simulink model "BasicACCTest"  (R2014a)
settings: Solver=ode45  StartTime=0.0  StopTime=10.0  RelTol=1e-3
values from neighbouring files (symbols this model uses):
  Engine =     [ECR1.mat]    (also in GenPT001.mat)
  Trans =     [ECR1.mat]    (also in GenPT001.mat)
libraries: simulink x2
settings Model: Creator=swami  LastModifiedBy=swami

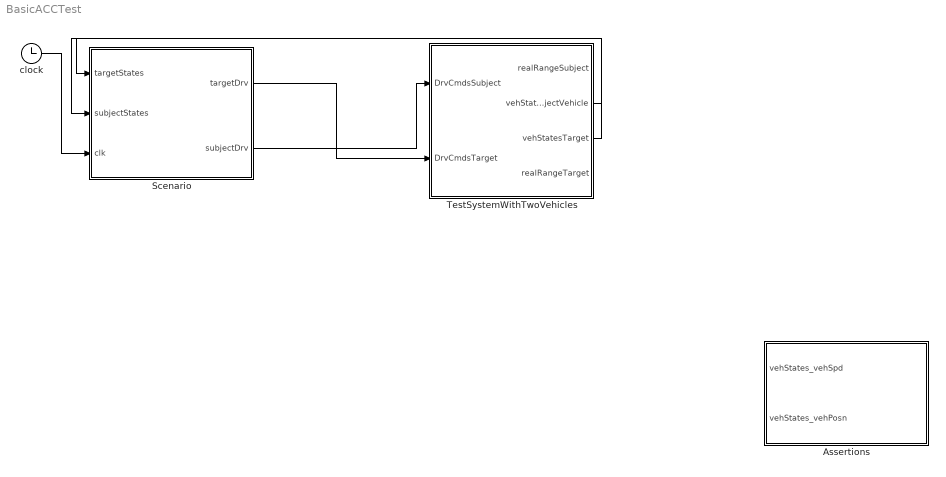
== system BasicACCTest ==
  Assertions : Subsystem
  Scenario : Stateflow chart  TreatAsAtomicUnit=on
  TestSystemWithTwoVehicles : Subsystem
  clock : Clock
  wires:
  Scenario/1(targetDrv) -> TestSystemWithTwoVehicles/2(DrvCmdsTarget)
  Scenario/2(subjectDrv) -> TestSystemWithTwoVehicles/1(DrvCmdsSubject)
  TestSystemWithTwoVehicles/3(vehStatesTarget) -> Scenario/1(targetStates)
  TestSystemWithTwoVehicles/2(vehStatesSubjectVehicle) -> Scenario/2(subjectStates)
  clock/1 -> Scenario/3(clk)

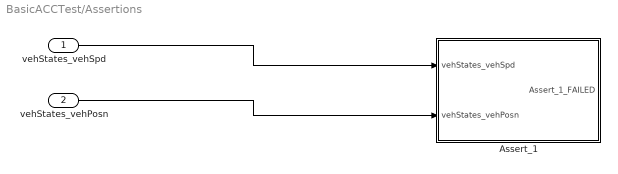
== system BasicACCTest/Assertions ==
  vehStates_vehSpd : Inport
  vehStates_vehPosn : Inport  Port=2
  Assert_1 : Subsystem
  wires:
  vehStates_vehSpd/1 -> Assert_1/1(vehStates_vehSpd)
  vehStates_vehPosn/1 -> Assert_1/2(vehStates_vehPosn)

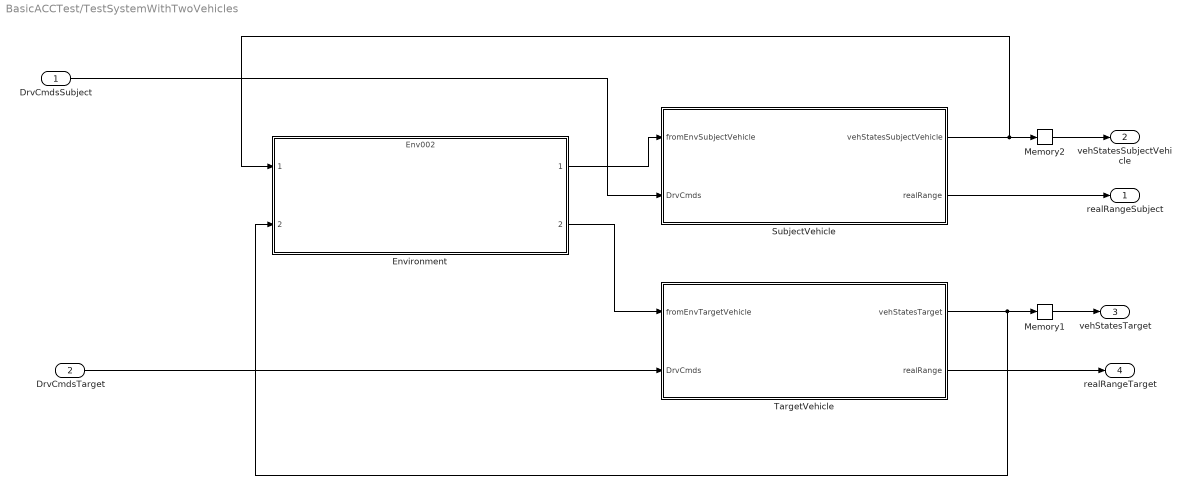
== system BasicACCTest/TestSystemWithTwoVehicles ==
  DrvCmdsSubject : Inport  OutDataTypeStr=double
  DrvCmdsTarget : Inport  Port=2
  Environment : ModelReference  ModelNameDialog=Env002  SimulationMode=Normal  Variant=on  OverrideUsingVariant=ECR1_varEnv002  ModelReferenceVersion=1.10  CopyOfModelName=Env002  DefaultDataLogging=on
      settings: AttributesFormatString=%<ActiveVariant>
  Memory1 : Memory
  Memory2 : Memory
  SubjectVehicle : Subsystem
  TargetVehicle : Subsystem
  realRangeSubject : Outport
  vehStatesSubjectVehicle : Outport  Port=2
  vehStatesTarget : Outport  Port=3
  realRangeTarget : Outport  Port=4
  wires:
  Memory1/1 -> vehStatesTarget/1
  Memory2/1 -> vehStatesSubjectVehicle/1
  DrvCmdsSubject/1 -> SubjectVehicle/2(DrvCmds)
  DrvCmdsTarget/1 -> TargetVehicle/2(DrvCmds)
  TargetVehicle/2(realRange) -> realRangeTarget/1
  SubjectVehicle/2(realRange) -> realRangeSubject/1
  SubjectVehicle/1(vehStatesSubjectVehicle) -> Memory2/1, Environment/1
  Environment/1 -> SubjectVehicle/1(fromEnvSubjectVehicle)
  Environment/2 -> TargetVehicle/1(fromEnvTargetVehicle)
  TargetVehicle/1(vehStatesTarget) -> Memory1/1, Environment/2

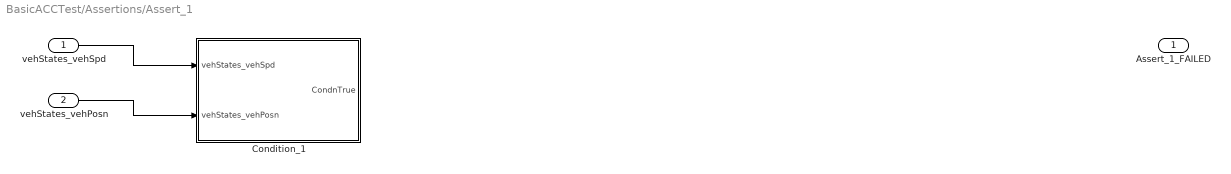
== system BasicACCTest/Assertions/Assert_1 ==
  vehStates_vehSpd : Inport
  vehStates_vehPosn : Inport  Port=2
  Condition_1 : Subsystem
  Assert_1_FAILED : Outport
  wires:
  vehStates_vehSpd/1 -> Condition_1/1(vehStates_vehSpd)
  vehStates_vehPosn/1 -> Condition_1/2(vehStates_vehPosn)

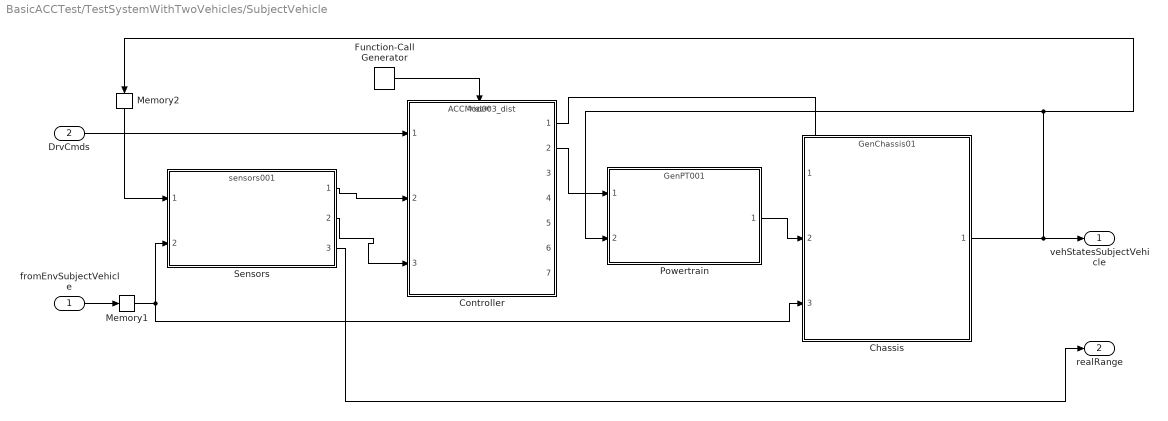
== system BasicACCTest/TestSystemWithTwoVehicles/SubjectVehicle ==
  fromEnvSubjectVehicle : Inport
  DrvCmds : Inport  Port=2
  Chassis : ModelReference  ModelNameDialog=GenChassis01  ParameterArgumentNames=Chassis  ParameterArgumentValues=ChassisSubject  SimulationMode=Normal  Variant=on  OverrideUsingVariant=ECR1_varChassis01  ModelReferenceVersion=1.19  CopyOfModelName=GenChassis01  DefaultDataLogging=on
      settings: AttributesFormatString=%<ActiveVariant>
  Controller : ModelReference  ModelNameDialog=ACCMod003_dist  ParameterArgumentNames=pACC  ParameterArgumentValues=pACCMod  Variant=on  OverrideUsingVariant=ECR1_varACCMod003_dist  ModelReferenceVersion=1.196  CopyOfModelName=ACCMod003_dist  DefaultDataLogging=on  TriggerPortName=Trigger  TriggerPortTriggerType=function-call  TriggerPortStatesWhenEnabling=held
      settings: AttributesFormatString=%<ActiveVariant>
  Function-Call Generator : simulink/Ports & Subsystems/Function-Call Generator  sample_time=0.1  numberOfIterations=1
  Memory1 : Memory
  Memory2 : Memory
  Powertrain : ModelReference  ModelNameDialog=GenPT001  ParameterArgumentNames=Trans,Engine  ParameterArgumentValues=Trans,Engine  SimulationMode=Normal  Variant=on  OverrideUsingVariant=ECR1_varGenPT001  ModelReferenceVersion=1.23  CopyOfModelName=GenPT001  DefaultDataLogging=on
      settings: AttributesFormatString=%<ActiveVariant>
  Sensors : ModelReference  ModelNameDialog=sensors001  SimulationMode=Normal  Variant=on  OverrideUsingVariant=ECR1_varSensor001  ModelReferenceVersion=1.21  CopyOfModelName=sensors001  DefaultDataLogging=on
      settings: AttributesFormatString=%<ActiveVariant>
  vehStatesSubjectVehicle : Outport
  realRange : Outport  Port=2
  wires:
  Sensors/3 -> realRange/1
  Function-Call Generator/1 -> Controller/Trigger
  Memory1/1 -> Chassis/3, Sensors/2
  fromEnvSubjectVehicle/1 -> Memory1/1
  Memory2/1 -> Sensors/1
  DrvCmds/1 -> Controller/1
  Sensors/2 -> Controller/3
  Sensors/1 -> Controller/2
  Controller/1 -> Chassis/1
  Powertrain/1 -> Chassis/2
  Controller/2 -> Powertrain/1
  Chassis/1 -> vehStatesSubjectVehicle/1, Powertrain/2, Memory2/1

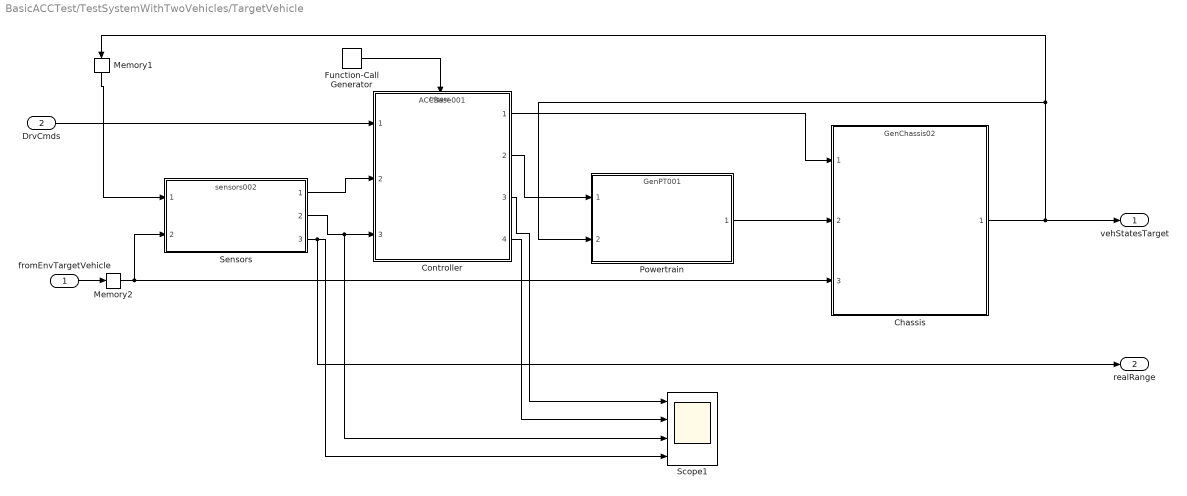
== system BasicACCTest/TestSystemWithTwoVehicles/TargetVehicle ==
  fromEnvTargetVehicle : Inport
  DrvCmds : Inport  Port=2
  Chassis : ModelReference  ModelNameDialog=GenChassis02  ParameterArgumentNames=Chassis  ParameterArgumentValues=ChassisTarget  SimulationMode=Normal  Variant=on  OverrideUsingVariant=ECR1_varChassis02  ModelReferenceVersion=1.19  CopyOfModelName=GenChassis02  DefaultDataLogging=on
      settings: AttributesFormatString=%<ActiveVariant>
  Controller : ModelReference  ModelNameDialog=ACCBase001  ParameterArgumentNames=pACC  ParameterArgumentValues=pACCBase  SimulationMode=Normal  Variant=on  OverrideUsingVariant=ECR1_var0005  ModelReferenceVersion=1.92  CopyOfModelName=ACCBase001  DefaultDataLogging=on  TriggerPortName=Trigger  TriggerPortTriggerType=function-call  TriggerPortStatesWhenEnabling=held
      settings: AttributesFormatString=%<ActiveVariant>
  Function-Call Generator : simulink/Ports & Subsystems/Function-Call Generator  sample_time=0.1  numberOfIterations=1
  Memory1 : Memory
  Memory2 : Memory
  Powertrain : ModelReference  ModelNameDialog=GenPT001  ParameterArgumentNames=Trans,Engine  ParameterArgumentValues=Trans,Engine  SimulationMode=Normal  Variant=on  OverrideUsingVariant=ECR1_varGenPT001  ModelReferenceVersion=1.23  CopyOfModelName=GenPT001  DefaultDataLogging=on
      settings: AttributesFormatString=%<ActiveVariant>
  Scope1 : Scope  NumInputPorts=4
  Sensors : ModelReference  ModelNameDialog=sensors002  SimulationMode=Normal  Variant=on  OverrideUsingVariant=varObject1  ModelReferenceVersion=1.19  CopyOfModelName=sensors002  DefaultDataLogging=on
      settings: AttributesFormatString=%<ActiveVariant>
  vehStatesTarget : Outport
  realRange : Outport  Port=2
  wires:
  Sensors/3 -> Scope1/4, realRange/1
  Controller/4 -> Scope1/2
  Controller/3 -> Scope1/1
  Function-Call Generator/1 -> Controller/Trigger
  Memory2/1 -> Chassis/3, Sensors/2
  Memory1/1 -> Sensors/1
  Chassis/1 -> Powertrain/2, Memory1/1, vehStatesTarget/1
  fromEnvTargetVehicle/1 -> Memory2/1
  Controller/2 -> Powertrain/1
  Powertrain/1 -> Chassis/2
  Controller/1 -> Chassis/1
  DrvCmds/1 -> Controller/1
  Sensors/1 -> Controller/2
  Sensors/2 -> Controller/3, Scope1/3

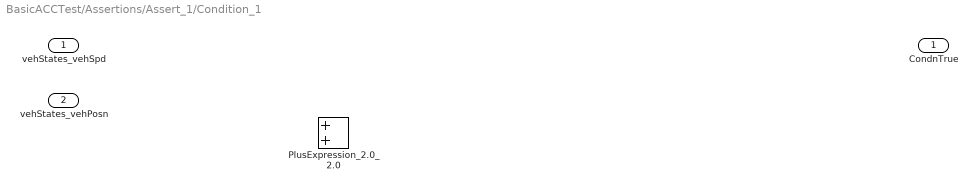
== system BasicACCTest/Assertions/Assert_1/Condition_1 ==
  vehStates_vehSpd : Inport
  vehStates_vehPosn : Inport  Port=2
  PlusExpression_2.0_2.0 : Sum
  CondnTrue : Outport

== stateflow chart BasicACCTest/Scenario ==
  state Act_TargetVehicle [parallel]
    settings: executionOrder=1
    state Act_TargetVehicle_Step1
    state Act_TargetVehicle_Step2
      state Act_TargetVehicle_Step2_1
        entry: targetDrv = [0,1,0,0];
      state Act_TargetVehicle_Step2_2
        entry: targetDrv = [0,0,1,50];
      (default) -> Act_TargetVehicle_Step2_1
      Act_TargetVehicle_Step2_1 -> Act_TargetVehicle_Step2_2 : [targetStates(2) >= 50]
    (default) -> Act_TargetVehicle_Step1
    Act_TargetVehicle_Step1 -> Act_TargetVehicle_Step2 : [clk > 0]
  state Act_SubjectVehicle [parallel]
    settings: executionOrder=2
    state Act_SubjectVehicle_Step1
    state Act_SubjectVehicle_Step2
      state Act_SubjectVehicle_Step2_1
        entry: subjectDrv = [0,1,0,0];
      state Act_SubjectVehicle_Step2_2
        entry: subjectDrv = [0,0,1,60];
      (default) -> Act_SubjectVehicle_Step2_1
      Act_SubjectVehicle_Step2_1 -> Act_SubjectVehicle_Step2_2 : [subjectStates(2) >= 60]
    (default) -> Act_SubjectVehicle_Step1
    Act_SubjectVehicle_Step1 -> Act_SubjectVehicle_Step2 : [clk > 0]
  data: targetStates input; subjectStates input; clk input; targetDrv output; subjectDrv output
